simulink model "group10"  (R2017b)
settings: Solver=VariableStepAuto  StartTime=0.0  StopTime=10.0  RelTol=1e-3
values from neighbouring files (symbols this model uses):
  den12 = [1 -1.94399066511 0.945546479969]    [Residual_generatorsQ2.mat]    (also in threeDiskOscillator_Q8.m = cell2mat(den1(2)); threeDiskOscillator_simData.m = cell2mat(den1(2)))
  den13 = [1 -1.94399066511 0.945546479969]    [Residual_generatorsQ2.mat]    (also in threeDiskOscillator_Q8.m = cell2mat(den1(3)); threeDiskOscillator_simData.m = cell2mat(den1(3)))
  den14 = [1 -1.94399066511 0.945546479969]    [Residual_generatorsQ2.mat]    (also in threeDiskOscillator_Q8.m = cell2mat(den1(4)); threeDiskOscillator_simData.m = cell2mat(den1(4)))
  den15 = [1 -1.94399066511 0.945546479969]    [Residual_generatorsQ2.mat]    (also in threeDiskOscillator_Q8.m = cell2mat(den1(5)); threeDiskOscillator_simData.m = cell2mat(den1(5)))
  den24 = [1 -1.94399066511 0.945546479969]    [Residual_generatorsQ2.mat]    (also in threeDiskOscillator_Q8.m = cell2mat(den2(4)); threeDiskOscillator_simData.m = cell2mat(den2(4)))
  den25 = [1 -1.94399066511 0.945546479969]    [Residual_generatorsQ2.mat]    (also in threeDiskOscillator_Q8.m = cell2mat(den2(5)); threeDiskOscillator_simData.m = cell2mat(den2(5)))
  h = 7.56835261331    [ECP_values_final.mat]    (also in Q2-5.mat; Residual_generators.mat = 0; Residual_generatorsQ2.mat; threeDiskOscillator_ALL.m = chi2inv(1 - P_F, 1)/2)
  J_2 = 0.00182883419357    [ECP_values_final.mat]    (also in Q2-5.mat; Residual_generators.mat; Residual_generatorsQ2.mat; threeDiskOscillator_ALL.m = ECP_values(2))
  J_3 = 0.00182883419357    [ECP_values_final.mat]    (also in Q2-5.mat; Residual_generators.mat; Residual_generatorsQ2.mat; threeDiskOscillator_ALL.m = ECP_values(3))
  k_1 = 2.78736928639    [ECP_values_final.mat]    (also in Q2-5.mat; Residual_generators.mat; Residual_generatorsQ2.mat; threeDiskOscillator_ALL.m = ECP_values(4))
  k_2 = 2.53389832968    [ECP_values_final.mat]    (also in Q2-5.mat; Residual_generators.mat; Residual_generatorsQ2.mat; threeDiskOscillator_ALL.m = ECP_values(5))
  M = 64    [ECP_values_final.mat]    (also in GLR_function.m = 25; Q2-5.mat = 265.152560978; Residual_generatorsQ2.mat = 1378.96164196; threeDiskOscillator_ALL.m = ceil(double(vpasolve([integral == P_D], [M], [0 200]))))
  mu_0 = 0    [ECP_values_final.mat]    (also in GLR.m; GLR_function.m; Q2-5.mat; Residual_generatorsQ2.mat)
  num12 = [0.212678500804 0.425357001609 0.212678500804]    [Residual_generatorsQ2.mat]    (also in threeDiskOscillator_Q8.m = cell2mat(num1(2)); threeDiskOscillator_simData.m = cell2mat(num1(2)))
  num13 = [0.592813521017 1.18562704203 0.592813521017]    [Residual_generatorsQ2.mat]    (also in threeDiskOscillator_Q8.m = cell2mat(num1(3)); threeDiskOscillator_simData.m = cell2mat(num1(3)))
  num14 = [-98.3875982708 192.213418816 -98.3526974211]    [Residual_generatorsQ2.mat]    (also in threeDiskOscillator_Q8.m = cell2mat(num1(4)); threeDiskOscillator_simData.m = cell2mat(num1(4)))
  num15 = [0.538905697947 1.07781139589 0.538905697947]    [Residual_generatorsQ2.mat]    (also in threeDiskOscillator_Q8.m = cell2mat(num1(5)); threeDiskOscillator_simData.m = cell2mat(num1(5)))
  num24 = [0.538905697947 1.07781139589 0.538905697947]    [Residual_generatorsQ2.mat]    (also in threeDiskOscillator_Q8.m = cell2mat(num2(4)); threeDiskOscillator_simData.m = cell2mat(num2(4)))
  num25 = [-97.7963881502 193.399045858 -97.7582804996]    [Residual_generatorsQ2.mat]    (also in threeDiskOscillator_Q8.m = cell2mat(num2(5)); threeDiskOscillator_simData.m = cell2mat(num2(5)))
  r_window = [0 0 0 0 0 0 0 0 0 0 0 0 ... (64 elements, 64x1)]    [ECP_values_final.mat]    (also in Residual_generatorsQ2.mat = [0 0 0 0 0 0 0 0 0 0 0 0 ... (1378 elements, 1378x1)]; threeDiskOscillator_ALL.m = zeros(M,1); threeDiskOscillator_Q6.m = zeros(floor(M),1); threeDiskOscillator_Q8.m = zeros(floor(M),1))
  sigma_c = 0.826228950229    [Residual_generatorsQ2.mat]    (also in threeDiskOscillator_Q8.m = double(Q_yr))
  T_s = 0.004    [ECP_values_final.mat]    (also in Q2-5.mat; Residual_generators.mat; Residual_generatorsQ2.mat; threeDiskOscillator_ALL.m)
settings Model: Creator=ECP502  LastModifiedBy=Administrator
settings SFSimCC: SimUseLocalCustomCode=on
settings RTWCC: RTWUseLocalCustomCode=on

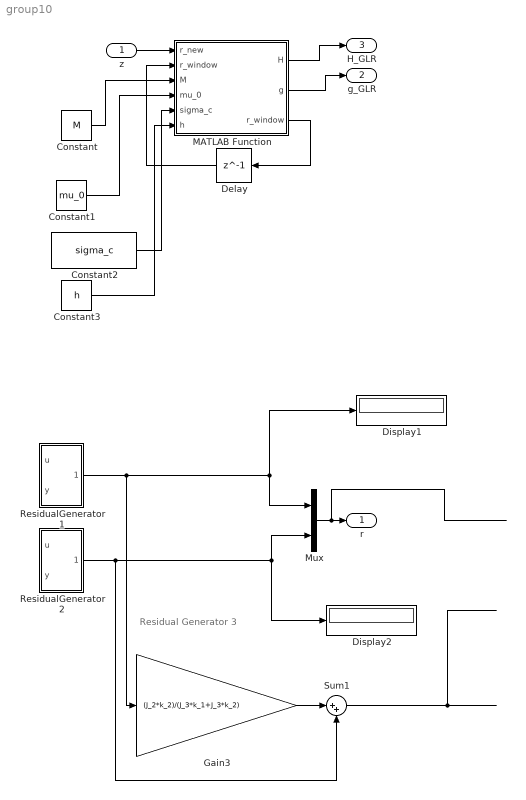
== system group10 ==
  note: Residual Generator 3
  z : Inport
  Constant : Constant  Value=M
  Constant1 : Constant  Value=mu_0
  Constant2 : Constant  Value=sigma_c
  Constant3 : Constant  Value=h
  Delay : Delay  DelayLength=1  InitialCondition=r_window  SampleTime=T_s
  Display1 : Display
  Display2 : Display
  Gain3 : Gain  Gain=(J_2*k_2)/(J_3*k_1+J_3*k_2)
  MATLAB Function : MATLAB Function  TreatAsAtomicUnit=on
  Mux : Mux  Inputs=2
  ResidualGenerator 1 : Subsystem
  ResidualGenerator 2 : Subsystem
  Sum1 : Sum  Inputs=|++
  r : Outport  VectorParamsAs1DForOutWhenUnconnected=off
  g_GLR : Outport  Port=2  VectorParamsAs1DForOutWhenUnconnected=off
  H_GLR : Outport  Port=3  VectorParamsAs1DForOutWhenUnconnected=off
  wires:
  Gain3/1 -> Sum1/1
  Sum1/1 -> ?
  ResidualGenerator 2/1(Out1) -> Mux/2, Display2/1, Sum1/2
  ? -> ResidualGenerator 2/1(u), ResidualGenerator 1/1(u)
  ? -> ResidualGenerator 1/2(y), ResidualGenerator 2/2(y)
  Mux/1 -> r/1
  ResidualGenerator 1/1(Out1) -> Display1/1, Mux/1, Gain3/1
  MATLAB Function/3(r_window) -> Delay/1
  Delay/1 -> MATLAB Function/2("r_window ")
  MATLAB Function/2(g) -> g_GLR/1
  MATLAB Function/1(H) -> H_GLR/1
  Constant2/1 -> MATLAB Function/5(sigma_c)
  Constant/1 -> MATLAB Function/3(M)
  Constant1/1 -> MATLAB Function/4(mu_0)
  Constant3/1 -> MATLAB Function/6(h)
  z/1 -> MATLAB Function/1(r_new)

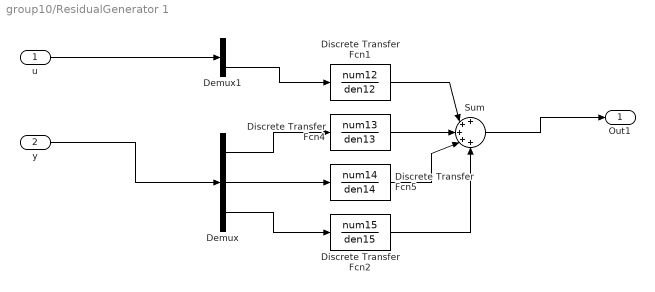
== system group10/ResidualGenerator 1 ==
  u : Inport
  y : Inport  Port=2
  Demux : Demux  Outputs=3
  Demux1 : Demux  Outputs=2
  Discrete Transfer Fcn1 : DiscreteTransferFcn  Numerator=num12  Denominator=den12
  Discrete Transfer Fcn2 : DiscreteTransferFcn  Numerator=num15  Denominator=den15
  Discrete Transfer Fcn4 : DiscreteTransferFcn  Numerator=num13  Denominator=den13
  Discrete Transfer Fcn5 : DiscreteTransferFcn  Numerator=num14  Denominator=den14
  Sum : Sum  Inputs=+++++
  Out1 : Outport
  wires:
  Demux/2 -> Discrete Transfer Fcn5/1
  Discrete Transfer Fcn5/1 -> Sum/4
  Sum/1 -> Out1/1
  Demux/1 -> Discrete Transfer Fcn4/1
  Demux/3 -> Discrete Transfer Fcn2/1
  Discrete Transfer Fcn1/1 -> Sum/2
  Discrete Transfer Fcn4/1 -> Sum/3
  Demux1/2 -> Discrete Transfer Fcn1/1
  Discrete Transfer Fcn2/1 -> Sum/5
  y/1 -> Demux/1
  u/1 -> Demux1/1

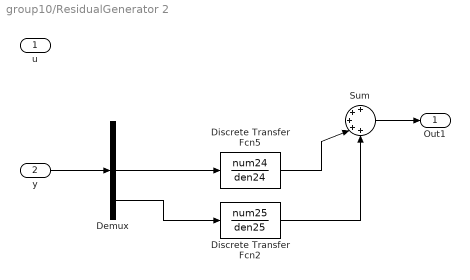
== system group10/ResidualGenerator 2 ==
  u : Inport
  y : Inport  Port=2
  Demux : Demux  Outputs=3
  Discrete Transfer Fcn2 : DiscreteTransferFcn  Numerator=num25  Denominator=den25
  Discrete Transfer Fcn5 : DiscreteTransferFcn  Numerator=num24  Denominator=den24
  Sum : Sum  Inputs=+++++
  Out1 : Outport
  wires:
  Demux/2 -> Discrete Transfer Fcn5/1
  Discrete Transfer Fcn5/1 -> Sum/4
  Sum/1 -> Out1/1
  Demux/3 -> Discrete Transfer Fcn2/1
  Discrete Transfer Fcn2/1 -> Sum/5
  y/1 -> Demux/1

== matlab function group10/MATLAB Function ==
  data: r_new input; H output; r_window input; g output; r_window output; M input; mu_0 input; sigma_c input; h input
function [H, g, r_window] = GLR(r_new, r_window, M, mu_0, sigma_c, h)

%sigma = 0.36229693539067544172329302373852;
%mu_0 = 0;
%M = 265;
%h=7.5684;

r_window = [r_window(2:end); r_new];


%Using equation 7.35 from the book

%calculating g from a running window.
g = 1/(2*sigma_c^2*M)*sum(r_window-mu_0)^2;

if (g > h)
    H = 1;
else
    H = 0;
end
